simulink model "nlmodel2019a"  (R2019a)
settings: Solver=ode45  StartTime=0.0  StopTime=10.0  RelTol=1e-3  EnableMultiTasking=on
values from neighbouring files (symbols this model uses):
  alpha1hat = 0.0114    [Linearize_whitebox.m]    (also in Linearize_whitebox_final.m; lqr_whitebox.mat; matrices.mat)
  area = 0.001    [nonlinid.m]
  boltz = 5.67e-8    (= 5.67e-08)    [Linearize_whitebox.m]    (also in Linearize_whitebox_final.m; lqr_whitebox.mat; matrices.mat; nonlinid.m)
  cphat = 501.9208    [Linearize_whitebox.m]    (also in Linearize_whitebox_final.m; lqr_whitebox.mat; matrices.mat)
  emis = 0.9    [nonlinid.m]
  m = 0.0052    [model.m]    (also in nonlinid.m = 0.004)
  Tamb = 18+273    (= 291)    [nonlinid.m]
  tau = 24.4408    [model.m]    (also in nonlinid.m = 24)
  uhat = 10.2021    [Linearize_whitebox.m]    (also in Linearize_whitebox_final.m; lqr_whitebox.mat; matrices.mat)
  x0 = [y1(1);y2(1)]    [Linearize_whitebox.m]    (also in Linearize_whitebox_final.m; lqr_whitebox.mat = [0 0]; matrices.mat = [293.042473118 292.064956012]; nonlinid.m)
settings Model: Creator=Eveline  LastModifiedBy=SIDTUDelft1
settings DataIOCC: LimitDataPoints=on  SaveFormat=Array  SignalLoggingSaveFormat=ModelDataLogs  ReturnWorkspaceOutputs=off
settings OptimizationCC: BooleanDataType=off
settings DebuggingCC: SaveWithParameterizedLinksMsg=none  UnderspecifiedInitializationDetection=Classic  MergeDetectMultiDrivingBlocksExec=none  SignalResolutionControl=TryResolveAllWithWarning  MultiTaskDSMMsg=warning  MultiTaskCondExecSysMsg=none
settings HardwareCC: TargetUnknown=on
settings ModelReferenceCC: PropagateSignalLabelsOutOfModel=off
settings GRTTargetCC: CombineOutputUpdateFcns=off  GRTInterface=on
settings ConfigComp: CovMetricSettings=dw  CovHtmlReporting=on

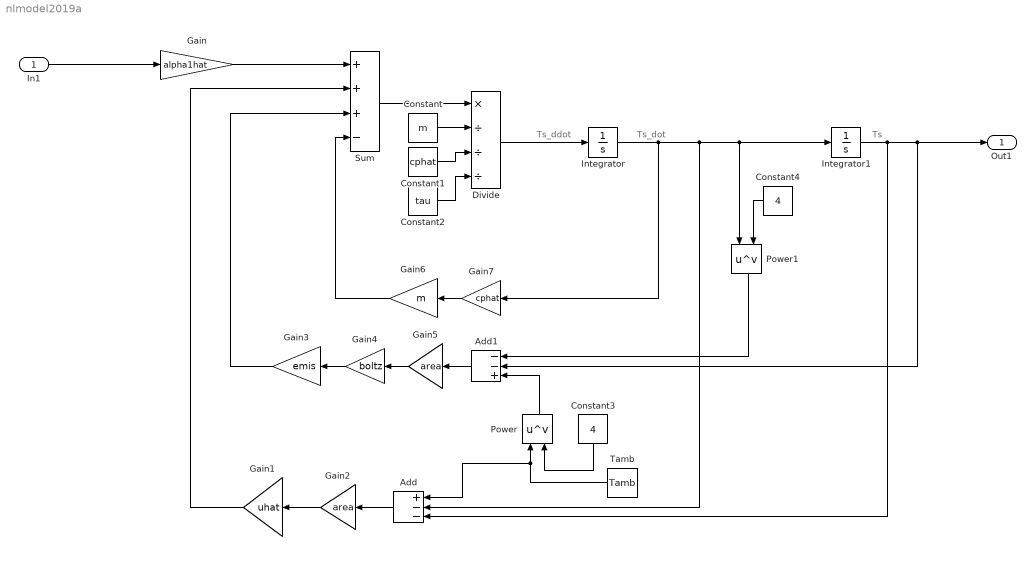
== system nlmodel2019a ==
  note: Ts_dot
  note: Ts_ddot
  note: Ts
  In1 : Inport
  Add : Sum  Inputs=+--
  Add1 : Sum  Inputs=--+
  Constant : Constant  Value=m
  Constant1 : Constant  Value=cphat
  Constant2 : Constant  Value=tau
  Constant3 : Constant  Value=4
  Constant4 : Constant  Value=4
  Divide : Product  Inputs=*///
  Gain : Gain  Gain=alpha1hat
  Gain1 : Gain  Gain=uhat
  Gain2 : Gain  Gain=area
  Gain3 : Gain  Gain=emis
  Gain4 : Gain  Gain=boltz
  Gain5 : Gain  Gain=area
  Gain6 : Gain  Gain=m
  Gain7 : Gain  Gain=cphat
  Integrator : Integrator  InitialCondition=x0(2)
  Integrator1 : Integrator  InitialCondition=x0(2)
  Power : Math  Operator=pow  SaturateOnIntegerOverflow=on
  Power1 : Math  Operator=pow  SaturateOnIntegerOverflow=on
  Sum : Sum  Inputs=+++-  SaturateOnIntegerOverflow=on
  Tamb : Constant  Value=Tamb
  Out1 : Outport
  wires:
  Integrator/1 -> Gain7/1, Add/2, Integrator1/1, Power1/1
  In1/1 -> Gain/1
  Gain1/1 -> Sum/2
  Integrator1/1 -> Add/3, Add1/2, Out1/1
  Constant/1 -> Divide/2
  Constant1/1 -> Divide/3
  Constant2/1 -> Divide/4
  Sum/1 -> Divide/1
  Divide/1 -> Integrator/1
  Gain/1 -> Sum/1
  Gain2/1 -> Gain1/1
  Add/1 -> Gain2/1
  Tamb/1 -> Power/1, Add/1
  Gain4/1 -> Gain3/1
  Gain5/1 -> Gain4/1
  Gain3/1 -> Sum/3
  Add1/1 -> Gain5/1
  Power/1 -> Add1/3
  Constant3/1 -> Power/2
  Constant4/1 -> Power1/2
  Power1/1 -> Add1/1
  Gain7/1 -> Gain6/1
  Gain6/1 -> Sum/4
